simulink model "Modello_Convertiplano"  (R2023b)
settings: Solver=VariableStepAuto  StartTime=0.0  StopTime=1000  RelTol=1e-3
values from neighbouring files (symbols this model uses):
  A_tot = [      A_att,         zeros(2,4) ... (first row only)    [LQG.m]
  B_tot = [B_att;  B_nom*D_att]    [LQG.m]
  C_tot = [D_nom*C_att,   C_nom]    [LQG.m]
  dq_0 = [0; 0]    [LQG.m]    (also in Programma_completo.m)
  Kc = - info.Kx    [LQG.m]
  Kc_int = -lqi(G, Q_z, R_u)    [LQG.m]
  Kf = info.L    [LQG.m]
  Km1 = 500    [LQG.m]    (also in Mix_sensitivity.m; Programma_completo.m; mu_synthesis.m = 10)
  Km2 = 100    [LQG.m]    (also in Mix_sensitivity.m = 100;.; Programma_completo.m; mu_synthesis.m = 20)
  q_0 = [2; -pi/18]    [LQG.m]    (also in Programma_completo.m = [0; 0])
  T1 = 0.5    [LQG.m]    (also in Mix_sensitivity.m; Programma_completo.m; mu_synthesis.m = 0.1)
  T2 = 0.5    [LQG.m]    (also in Mix_sensitivity.m; Programma_completo.m; mu_synthesis.m = 0.2)
  Tm1 = 5    [LQG.m]    (also in Mix_sensitivity.m; Programma_completo.m; mu_synthesis.m)
  Tm2 = 5    [LQG.m]    (also in Mix_sensitivity.m; Programma_completo.m; mu_synthesis.m)
settings Model: Creator=lucag  LastModifiedBy=jacoc

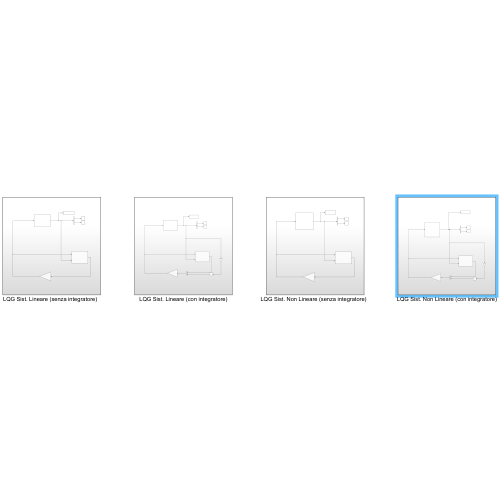
[thumbnail: Simulink's stored preview of the top-level diagram]
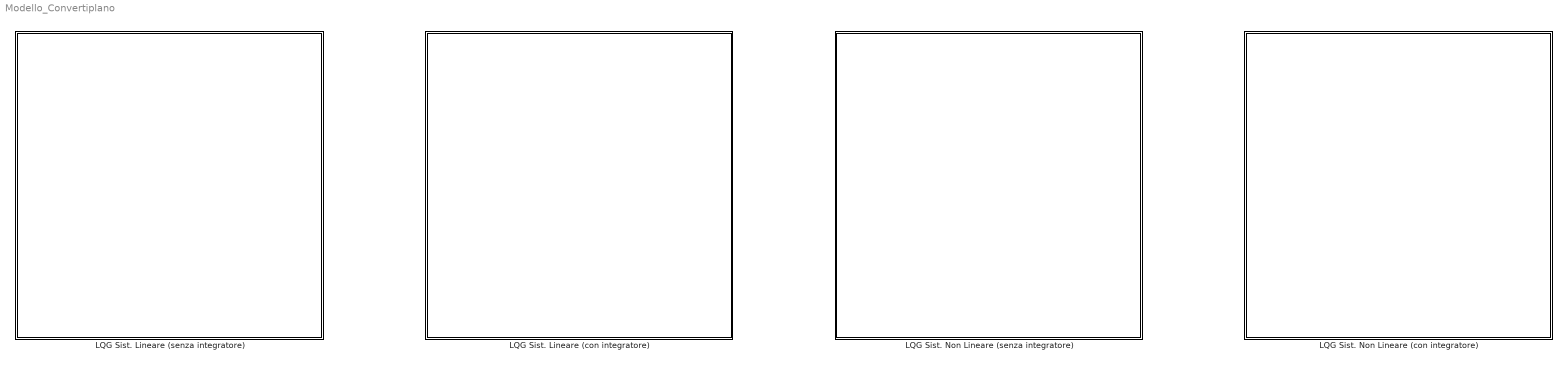
== system Modello_Convertiplano ==
  LQG Sist. Lineare (con integratore) : Subsystem
  "LQG Sist. Lineare (senza integratore)  " : Subsystem
  LQG Sist. Non Lineare (con integratore) : Subsystem
  "LQG Sist. Non Lineare (senza integratore)  " : Subsystem

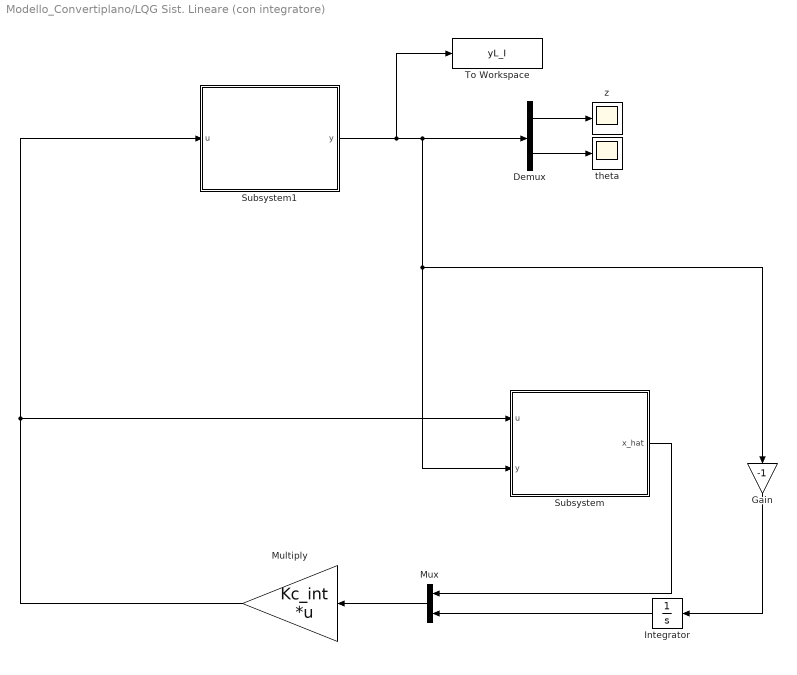
== system Modello_Convertiplano/LQG Sist. Lineare (con integratore) ==
  Demux : Demux  Outputs=2
  Gain : Gain  Gain=-1
  Integrator : Integrator  InitialCondition=[0;0]
  Multiply : Gain  Gain=Kc_int  Multiplication=Matrix(K*u) (u vector)
  Mux : Mux  Inputs=2
  Subsystem : Subsystem
  Subsystem1 : Subsystem
  To Workspace : ToWorkspace  VariableName=yL_I  SaveFormat=Timeseries  SampleTime=-1
  theta : Scope
  z : Scope
  wires:
  Demux/2 -> theta/1
  Multiply/1 -> Subsystem/1(u), Subsystem1/1(u)
  Demux/1 -> z/1
  Subsystem1/1(y) -> To Workspace/1, Demux/1, Gain/1, Subsystem/2(y)
  Mux/1 -> Multiply/1
  Subsystem/1(x_hat) -> Mux/1
  Gain/1 -> Integrator/1
  Integrator/1 -> Mux/2

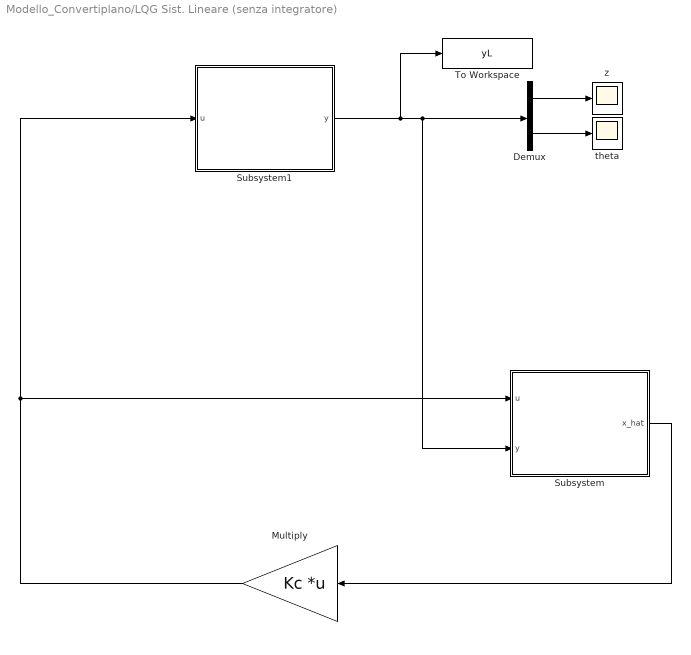
== system Modello_Convertiplano/LQG Sist. Lineare (senza integratore)   ==
  Demux : Demux  Outputs=2
  Multiply : Gain  Gain=Kc  Multiplication=Matrix(K*u) (u vector)
  Subsystem : Subsystem
  Subsystem1 : Subsystem
  To Workspace : ToWorkspace  VariableName=yL  SaveFormat=Timeseries  SampleTime=-1
  theta : Scope
  z : Scope
  wires:
  Subsystem1/1(y) -> To Workspace/1, Subsystem/2(y), Demux/1
  Demux/1 -> z/1
  Multiply/1 -> Subsystem1/1(u), Subsystem/1(u)
  Demux/2 -> theta/1
  Subsystem/1(x_hat) -> Multiply/1

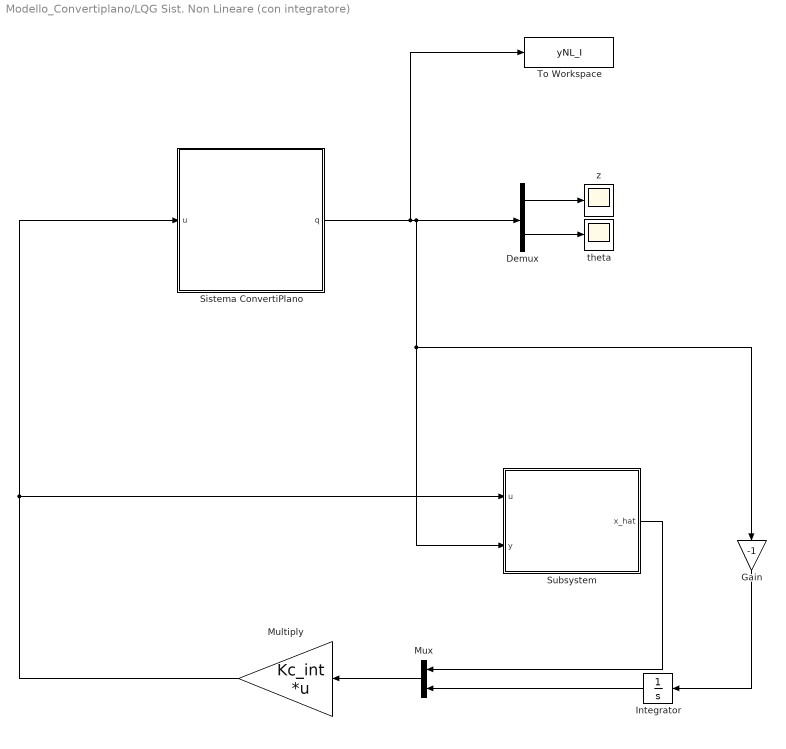
== system Modello_Convertiplano/LQG Sist. Non Lineare (con integratore) ==
  Demux : Demux  Outputs=2
  Gain : Gain  Gain=-1
  Integrator : Integrator  InitialCondition=[0;0]
  Multiply : Gain  Gain=Kc_int  Multiplication=Matrix(K*u) (u vector)
  Mux : Mux  Inputs=2
  Sistema ConvertiPlano : Subsystem
  Subsystem : Subsystem
  To Workspace : ToWorkspace  VariableName=yNL_I  SaveFormat=Timeseries  SampleTime=-1
  theta : Scope
  z : Scope
  wires:
  Integrator/1 -> Mux/2
  Gain/1 -> Integrator/1
  Subsystem/1(x_hat) -> Mux/1
  Mux/1 -> Multiply/1
  Sistema ConvertiPlano/1(q) -> To Workspace/1, Subsystem/2(y), Gain/1, Demux/1
  Demux/1 -> z/1
  Multiply/1 -> Sistema ConvertiPlano/1(u), Subsystem/1(u)
  Demux/2 -> theta/1

== system Modello_Convertiplano/LQG Sist. Non Lineare (senza integratore)   ==
  Demux : Demux  Outputs=2
  Multiply : Gain  Gain=Kc  Multiplication=Matrix(K*u) (u vector)
  Sistema ConvertiPlano : Subsystem
  Subsystem1 : Subsystem
  To Workspace : ToWorkspace  VariableName=yNL  SaveFormat=Timeseries  SampleTime=-1
  theta : Scope
  z : Scope
  wires:
  Subsystem1/1(x_hat) -> Multiply/1
  Demux/2 -> theta/1
  Multiply/1 -> Subsystem1/1(u), Sistema ConvertiPlano/1(u)
  Demux/1 -> z/1
  Sistema ConvertiPlano/1(q) -> To Workspace/1, Subsystem1/2(y), Demux/1

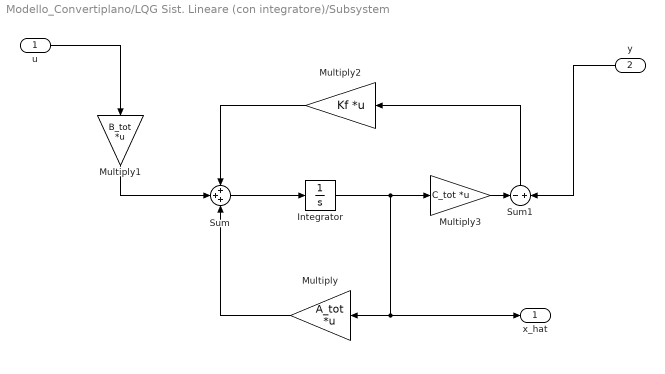
== system Modello_Convertiplano/LQG Sist. Lineare (con integratore)/Subsystem ==
  u : Inport
  y : Inport  Port=2
  Integrator : Integrator  InitialCondition=[0; 0; 0; 0; 0; 0]
  Multiply : Gain  Gain=A_tot  Multiplication=Matrix(K*u) (u vector)
  Multiply1 : Gain  Gain=B_tot  Multiplication=Matrix(K*u) (u vector)
  Multiply2 : Gain  Gain=Kf  Multiplication=Matrix(K*u) (u vector)
  Multiply3 : Gain  Gain=C_tot  Multiplication=Matrix(K*u) (u vector)
  Sum : Sum  Inputs=+++
  Sum1 : Sum  Inputs=-+
  x_hat : Outport
  wires:
  y/1 -> Sum1/2
  Integrator/1 -> Multiply3/1, Multiply/1, x_hat/1
  u/1 -> Multiply1/1
  Multiply1/1 -> Sum/2
  Multiply2/1 -> Sum/1
  Multiply/1 -> Sum/3
  Sum1/1 -> Multiply2/1
  Sum/1 -> Integrator/1
  Multiply3/1 -> Sum1/1

== system Modello_Convertiplano/LQG Sist. Lineare (con integratore)/Subsystem1 ==
  u : Inport
  Integrator : Integrator  InitialCondition=[0; 0; dq_0; q_0]
  Multiply : Gain  Gain=A_tot  Multiplication=Matrix(K*u) (u vector)
  Multiply1 : Gain  Gain=B_tot  Multiplication=Matrix(K*u) (u vector)
  Multiply3 : Gain  Gain=C_tot  Multiplication=Matrix(K*u) (u vector)
  Sum : Sum  Inputs=|++
  y : Outport
  wires:
  Multiply/1 -> Sum/2
  Multiply1/1 -> Sum/1
  Sum/1 -> Integrator/1
  Multiply3/1 -> y/1
  u/1 -> Multiply1/1
  Integrator/1 -> Multiply/1, Multiply3/1

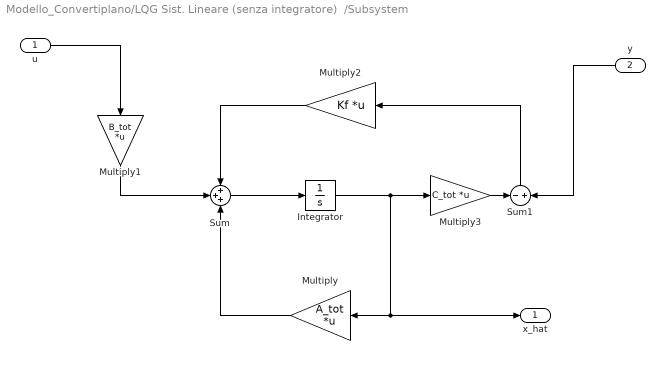
== system Modello_Convertiplano/LQG Sist. Lineare (senza integratore)  /Subsystem ==
  u : Inport
  y : Inport  Port=2
  Integrator : Integrator  InitialCondition=[0; 0; 0; 0; 0; 0]
  Multiply : Gain  Gain=A_tot  Multiplication=Matrix(K*u) (u vector)
  Multiply1 : Gain  Gain=B_tot  Multiplication=Matrix(K*u) (u vector)
  Multiply2 : Gain  Gain=Kf  Multiplication=Matrix(K*u) (u vector)
  Multiply3 : Gain  Gain=C_tot  Multiplication=Matrix(K*u) (u vector)
  Sum : Sum  Inputs=+++
  Sum1 : Sum  Inputs=-+
  x_hat : Outport
  wires:
  Multiply3/1 -> Sum1/1
  Sum/1 -> Integrator/1
  Sum1/1 -> Multiply2/1
  Multiply/1 -> Sum/3
  Multiply2/1 -> Sum/1
  Multiply1/1 -> Sum/2
  u/1 -> Multiply1/1
  Integrator/1 -> x_hat/1, Multiply/1, Multiply3/1
  y/1 -> Sum1/2

== system Modello_Convertiplano/LQG Sist. Lineare (senza integratore)  /Subsystem1 ==
  u : Inport
  Integrator : Integrator  InitialCondition=[0; 0; dq_0; q_0]
  Multiply : Gain  Gain=A_tot  Multiplication=Matrix(K*u) (u vector)
  Multiply1 : Gain  Gain=B_tot  Multiplication=Matrix(K*u) (u vector)
  Multiply3 : Gain  Gain=C_tot  Multiplication=Matrix(K*u) (u vector)
  Sum : Sum  Inputs=|++
  y : Outport
  wires:
  Integrator/1 -> Multiply3/1, Multiply/1
  u/1 -> Multiply1/1
  Multiply3/1 -> y/1
  Sum/1 -> Integrator/1
  Multiply1/1 -> Sum/1
  Multiply/1 -> Sum/2

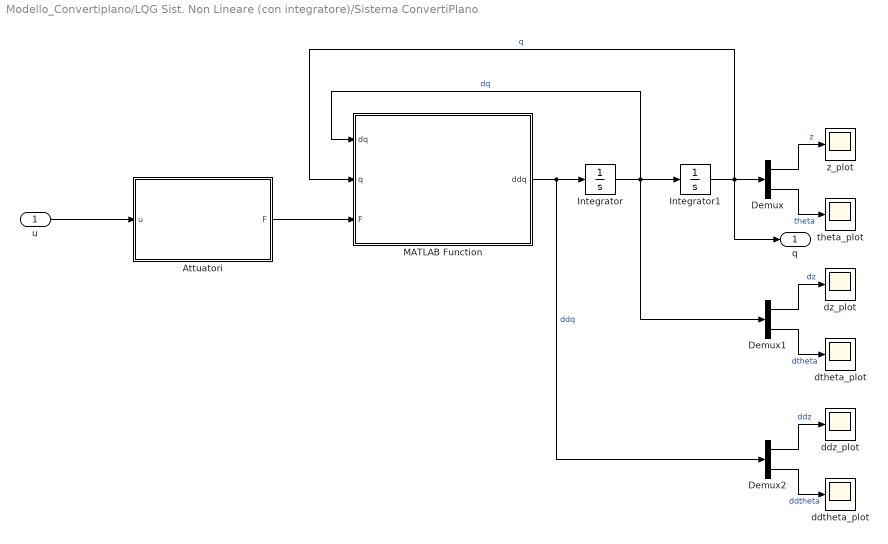
== system Modello_Convertiplano/LQG Sist. Non Lineare (con integratore)/Sistema ConvertiPlano ==
  u : Inport
  Attuatori : Subsystem
  Demux : Demux  Outputs=2
  Demux1 : Demux  Outputs=2
  Demux2 : Demux  Outputs=2
  Integrator : Integrator  InitialCondition=dq_0
  Integrator1 : Integrator  InitialCondition=q_0
  MATLAB Function : MATLAB Function  TreatAsAtomicUnit=on
  ddtheta_plot : Scope
  ddz_plot : Scope
  dtheta_plot : Scope
  dz_plot : Scope
  theta_plot : Scope
  z_plot : Scope
  q : Outport
  wires:
  Integrator1/1 -> q/1, Demux/1, MATLAB Function/2(q)  "q"
  Demux/2 -> theta_plot/1  "theta"
  Demux2/1 -> ddz_plot/1  "ddz"
  Demux/1 -> z_plot/1  "z"
  Integrator/1 -> Demux1/1, MATLAB Function/1(dq), Integrator1/1  "dq"
  Demux1/2 -> dtheta_plot/1  "dtheta"
  MATLAB Function/1(ddq) -> Demux2/1, Integrator/1  "ddq"
  Demux2/2 -> ddtheta_plot/1  "ddtheta"
  Demux1/1 -> dz_plot/1  "dz"
  u/1 -> Attuatori/1(u)
  Attuatori/1(F) -> MATLAB Function/3(F)

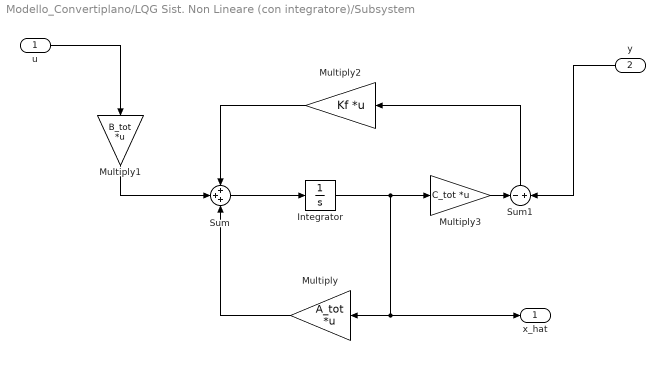
== system Modello_Convertiplano/LQG Sist. Non Lineare (con integratore)/Subsystem ==
  u : Inport
  y : Inport  Port=2
  Integrator : Integrator  InitialCondition=[0; 0; 0; 0; 0; 0]
  Multiply : Gain  Gain=A_tot  Multiplication=Matrix(K*u) (u vector)
  Multiply1 : Gain  Gain=B_tot  Multiplication=Matrix(K*u) (u vector)
  Multiply2 : Gain  Gain=Kf  Multiplication=Matrix(K*u) (u vector)
  Multiply3 : Gain  Gain=C_tot  Multiplication=Matrix(K*u) (u vector)
  Sum : Sum  Inputs=+++
  Sum1 : Sum  Inputs=-+
  x_hat : Outport
  wires:
  Multiply3/1 -> Sum1/1
  Sum/1 -> Integrator/1
  Sum1/1 -> Multiply2/1
  Multiply/1 -> Sum/3
  Multiply2/1 -> Sum/1
  Multiply1/1 -> Sum/2
  u/1 -> Multiply1/1
  Integrator/1 -> x_hat/1, Multiply/1, Multiply3/1
  y/1 -> Sum1/2

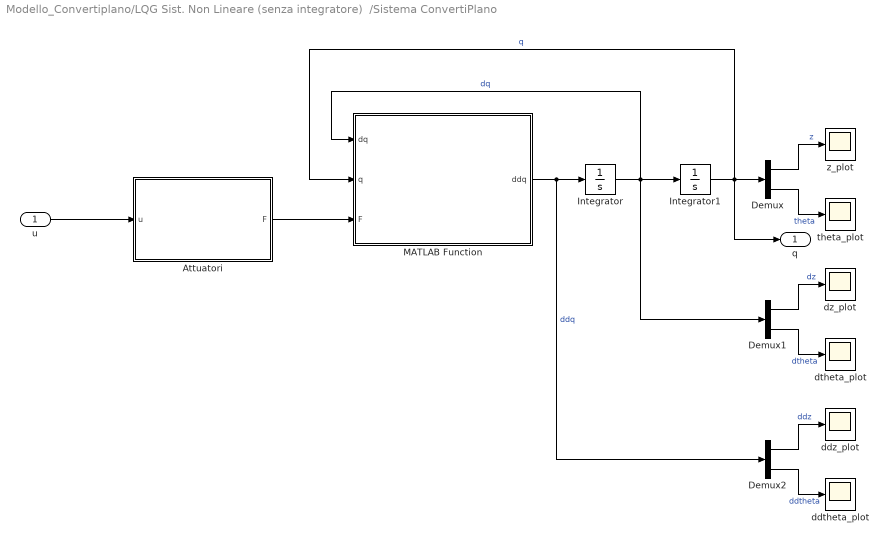
== system Modello_Convertiplano/LQG Sist. Non Lineare (senza integratore)  /Sistema ConvertiPlano ==
  u : Inport
  Attuatori : Subsystem
  Demux : Demux  Outputs=2
  Demux1 : Demux  Outputs=2
  Demux2 : Demux  Outputs=2
  Integrator : Integrator  InitialCondition=dq_0
  Integrator1 : Integrator  InitialCondition=q_0
  MATLAB Function : MATLAB Function  TreatAsAtomicUnit=on
  ddtheta_plot : Scope
  ddz_plot : Scope
  dtheta_plot : Scope
  dz_plot : Scope
  theta_plot : Scope
  z_plot : Scope
  q : Outport
  wires:
  Integrator1/1 -> q/1, Demux/1, MATLAB Function/2(q)  "q"
  Demux/2 -> theta_plot/1  "theta"
  Demux2/1 -> ddz_plot/1  "ddz"
  Demux/1 -> z_plot/1  "z"
  Integrator/1 -> Demux1/1, MATLAB Function/1(dq), Integrator1/1  "dq"
  Demux1/2 -> dtheta_plot/1  "dtheta"
  MATLAB Function/1(ddq) -> Demux2/1, Integrator/1  "ddq"
  Demux2/2 -> ddtheta_plot/1  "ddtheta"
  Demux1/1 -> dz_plot/1  "dz"
  u/1 -> Attuatori/1(u)
  Attuatori/1(F) -> MATLAB Function/3(F)

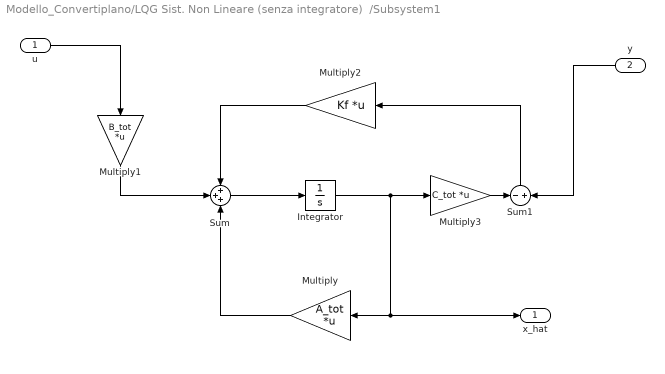
== system Modello_Convertiplano/LQG Sist. Non Lineare (senza integratore)  /Subsystem1 ==
  u : Inport
  y : Inport  Port=2
  Integrator : Integrator  InitialCondition=[0; 0; 0; 0; 0; 0]
  Multiply : Gain  Gain=A_tot  Multiplication=Matrix(K*u) (u vector)
  Multiply1 : Gain  Gain=B_tot  Multiplication=Matrix(K*u) (u vector)
  Multiply2 : Gain  Gain=Kf  Multiplication=Matrix(K*u) (u vector)
  Multiply3 : Gain  Gain=C_tot  Multiplication=Matrix(K*u) (u vector)
  Sum : Sum  Inputs=+++
  Sum1 : Sum  Inputs=-+
  x_hat : Outport
  wires:
  Multiply3/1 -> Sum1/1
  Sum/1 -> Integrator/1
  Sum1/1 -> Multiply2/1
  Multiply/1 -> Sum/3
  Multiply2/1 -> Sum/1
  Multiply1/1 -> Sum/2
  u/1 -> Multiply1/1
  Integrator/1 -> x_hat/1, Multiply/1, Multiply3/1
  y/1 -> Sum1/2

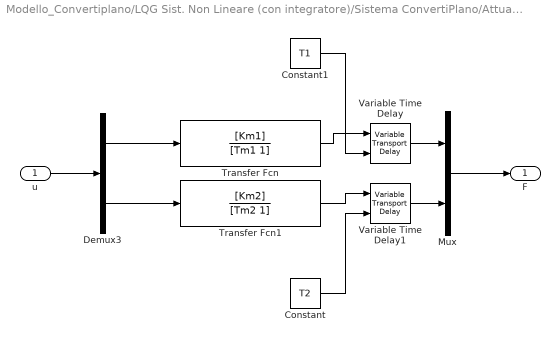
== system Modello_Convertiplano/LQG Sist. Non Lineare (con integratore)/Sistema ConvertiPlano/Attuatori ==
  u : Inport
  Constant : Constant  Value=T2
  Constant1 : Constant  Value=T1
  Demux3 : Demux  Outputs=2
  Mux : Mux  Inputs=2
  Transfer Fcn : TransferFcn  Numerator=[Km1]  Denominator=[Tm1 1]
  Transfer Fcn1 : TransferFcn  Numerator=[Km2]  Denominator=[Tm2 1]
  Variable Time Delay : VariableTransportDelay  MaximumDelay=10  PadeOrder=1
  Variable Time Delay1 : VariableTransportDelay  MaximumDelay=10  PadeOrder=1
  F : Outport
  wires:
  u/1 -> Demux3/1
  Demux3/1 -> Transfer Fcn/1
  Demux3/2 -> Transfer Fcn1/1
  Mux/1 -> F/1
  Variable Time Delay1/1 -> Mux/2
  Variable Time Delay/1 -> Mux/1
  Constant1/1 -> Variable Time Delay/2
  Transfer Fcn/1 -> Variable Time Delay/1
  Transfer Fcn1/1 -> Variable Time Delay1/1
  Constant/1 -> Variable Time Delay1/2

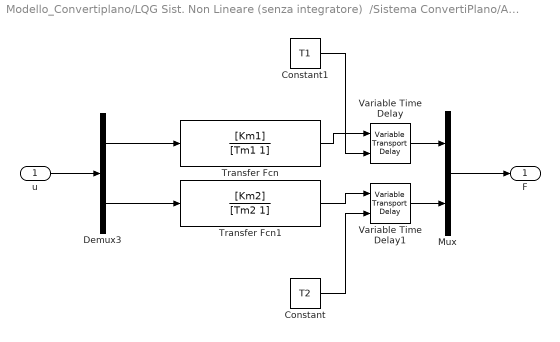
== system Modello_Convertiplano/LQG Sist. Non Lineare (senza integratore)  /Sistema ConvertiPlano/Attuatori ==
  u : Inport
  Constant : Constant  Value=T2
  Constant1 : Constant  Value=T1
  Demux3 : Demux  Outputs=2
  Mux : Mux  Inputs=2
  Transfer Fcn : TransferFcn  Numerator=[Km1]  Denominator=[Tm1 1]
  Transfer Fcn1 : TransferFcn  Numerator=[Km2]  Denominator=[Tm2 1]
  Variable Time Delay : VariableTransportDelay  MaximumDelay=10  PadeOrder=1
  Variable Time Delay1 : VariableTransportDelay  MaximumDelay=10  PadeOrder=1
  F : Outport
  wires:
  u/1 -> Demux3/1
  Demux3/1 -> Transfer Fcn/1
  Demux3/2 -> Transfer Fcn1/1
  Mux/1 -> F/1
  Variable Time Delay1/1 -> Mux/2
  Variable Time Delay/1 -> Mux/1
  Constant1/1 -> Variable Time Delay/2
  Transfer Fcn/1 -> Variable Time Delay/1
  Transfer Fcn1/1 -> Variable Time Delay1/1
  Constant/1 -> Variable Time Delay1/2

== matlab function Modello_Convertiplano/LQG Sist. Non Lineare (senza integratore)  /Sistema ConvertiPlano/MATLAB Function ==
  settings: updateMethod=CONTINUOUS
  data: dq input; ddq output; q input; F input; params_plano parameter
function ddq = ModelloDinamicoAereo(dq, q, F, params_plano)

    % Variabili di Stato %
    dz = dq(1);
    dtheta = dq(2);

    z = q(1);
    theta = q(2);
    
    % Ingressi %
    f_m = F(1);
    f_a = F(2);

    % Parametri fisici (con incertezza)
    J = params_plano(1);
    m = params_plano(2);
    b = params_plano(3);
    beta = params_plano(4);
    l = params_plano(5);

    g = params_plano(6);

    % Equazioni del modello fisico %
    ddz = -b/m * dz + f_m/m * cos(theta) - g;
    ddtheta = -beta/J * dtheta + 2*l/J * f_a;

    ddq = [ddz; ddtheta];

end

== matlab function Modello_Convertiplano/LQG Sist. Non Lineare (con integratore)/Sistema ConvertiPlano/MATLAB Function ==
  settings: updateMethod=CONTINUOUS
  data: dq input; ddq output; q input; F input; params_plano parameter
function ddq = ModelloDinamicoAereo(dq, q, F, params_plano)

    % Variabili di Stato %
    dz = dq(1);
    dtheta = dq(2);

    z = q(1);
    theta = q(2);
    
    % Ingressi %
    f_m = F(1);
    f_a = F(2);

    % Parametri fisici (con incertezza)
    J = params_plano(1);
    m = params_plano(2);
    b = params_plano(3);
    beta = params_plano(4);
    l = params_plano(5);

    g = params_plano(6);

    % Equazioni del modello fisico %
    ddz = -b/m * dz + f_m/m * cos(theta) - g;
    ddtheta = -beta/J * dtheta + 2*l/J * f_a;

    ddq = [ddz; ddtheta];

end
